simulink subsystem "baro_processing"  (R2024b)
settings: Solver=VariableStepAuto  StartTime=0.0  StopTime=10.0  RelTol=1e-3
undefined symbols (not defined in the file or in its folder): controller_rate, GROUND_LEVEL
libraries: simulink x1
settings Model: Creator=yevge  LastModifiedBy=yevge

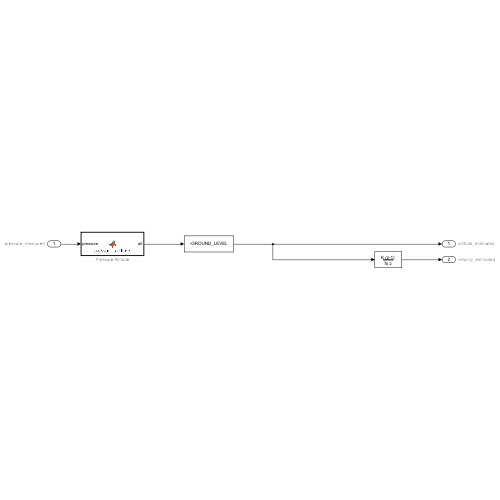
[thumbnail: Simulink's stored preview of the top-level diagram]
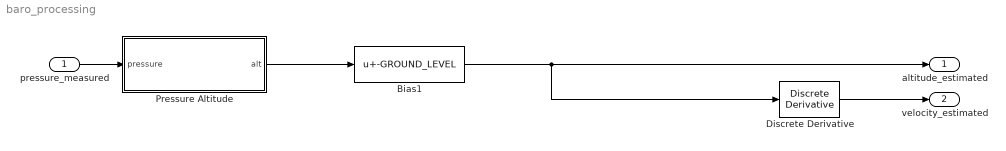
== system baro_processing ==
  pressure_measured : Inport  Unit=Pa  PortDimensions=1
  Bias1 : Bias  Bias=-GROUND_LEVEL  SaturateOnIntegerOverflow=off
  Discrete Derivative : simulink/Discrete/Discrete Derivative  gainval=1.0  ICPrevScaledInput=0.0  OutMin=[]  OutMax=[]  OutDataType=fixdt(1, 16)  OutScaling=2^-10  DoSatur=off
  Pressure Altitude : MATLAB Function  TreatAsAtomicUnit=on
  altitude_estimated : Outport  Unit=m  PortDimensions=1  SampleTime=1/controller_rate
  velocity_estimated : Outport  Port=2  Unit=m/s  PortDimensions=1  SampleTime=1/controller_rate
  wires:
  Discrete Derivative/1 -> velocity_estimated/1
  pressure_measured/1 -> Pressure Altitude/1(pressure)
  Pressure Altitude/1(alt) -> Bias1/1
  Bias1/1 -> Discrete Derivative/1, altitude_estimated/1

== matlab function baro_processing/Pressure Altitude ==
  data: pressure input; alt output
function alt = pressure_altitude(pressure)
    alt = (1 - (pressure ./ 101325).^(0.190284)) .* 145366.45 * 0.3048;
end
